simulink model "simulation_overall_1"  (R2024b)
settings: Solver=VariableStepAuto  StartTime=0.0  StopTime=10  MaxStep=1e-3  RelTol=1e-5
values from neighbouring files (symbols this model uses):
  dd_cable_len = diff(diff_cable_len)/dTheta    [sim_setup_1.m]
  del_theta = beam_defl    [sim_setup.m]    (also in sim_setup_1.m)
  del_theta0 = const.init_deflection    [sim_setup.m]    (also in sim_setup_1.m)
  diff_cable_len = diff(cable_len)/dTheta    [sim_setup_1.m]
  diff_del = diff(del_theta)/dTheta    [sim_setup.m]    (also in sim_setup_1.m)
  J = 0.0001    [sim_setup.m]    (also in sim_setup_1.m = 9.466956e-05)
  Jm = 32*1e-7    (= 3.2e-06)    [sim_setup_1.m]
  Jw = 12778*1e-9    (= 1.2778e-05)    [sim_setup_1.m]
  k = const.beam_stiffness    [sim_setup.m]    (also in sim_setup_1.m)
  Kt = 0.13    [sim_setup_1.m]
  N = 8    [sim_setup_1.m]
  R = 32e-3    (= 0.032)    [sim_setup_1.m]
  Sat_angle_max = ang(end)    [sim_setup_1.m]
  Sat_angle_min = ang(1)    [sim_setup_1.m]
  Sat_force_max = force(end)    [sim_setup_1.m]
  Sat_force_min = force(1)    [sim_setup_1.m]
  T_ang = ang(1:length(ang)-1)    [sim_setup.m]    (also in sim_setup_1.m)
undefined symbols (not defined in the file or in its folder): ang, cable_len
libraries: slpidlib x2, simulink_extras x1, simulink x1
settings Model: Creator=HNGG  LastModifiedBy=divg2
settings OptimizationCC: ReuseModelBlockBuffer=off
settings RTWCC: GPUComputeCapability=3.5

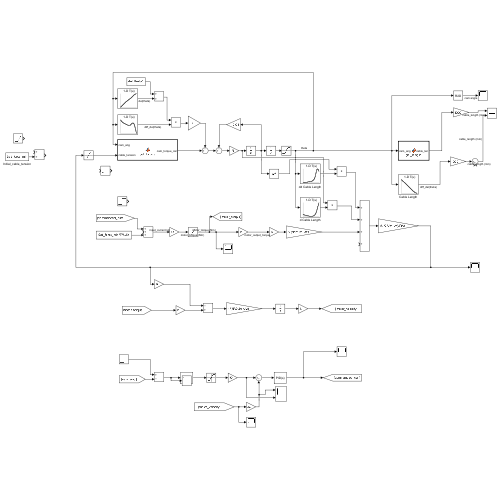
[thumbnail: Simulink's stored preview of the top-level diagram]
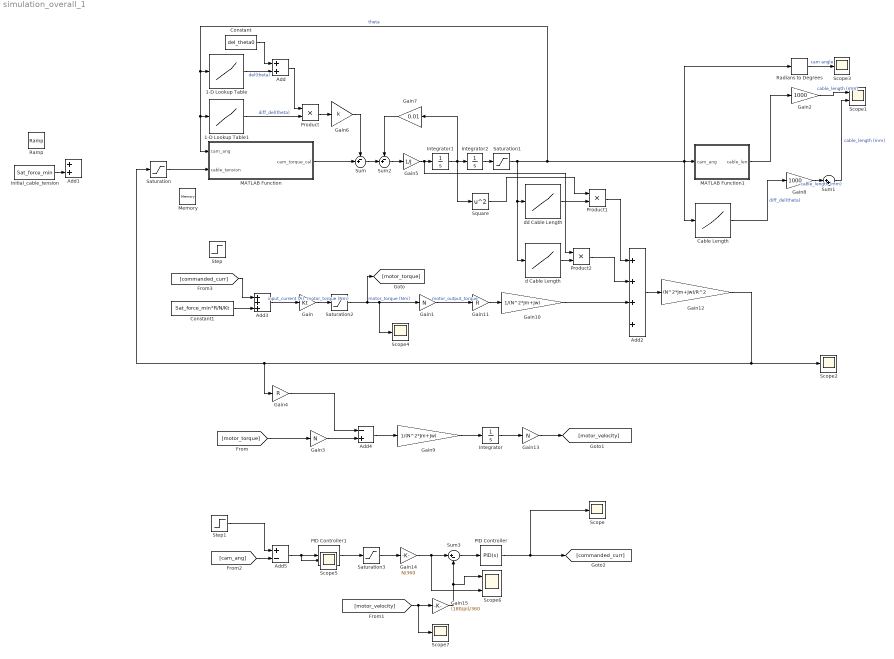
== system simulation_overall_1 ==
  1-D Lookup Table : Lookup_n-D  NumberOfTableDimensions=1  BreakpointsForDimension1=ang  Table=del_theta  InternalRulePriority=Speed  RndMeth=Simplest
  1-D Lookup Table1 : Lookup_n-D  NumberOfTableDimensions=1  BreakpointsForDimension1=T_ang  Table=diff_del  InternalRulePriority=Speed  RndMeth=Simplest
  Add : Sum
  Add1 : Sum
  Add2 : Sum  Inputs=++++
  Add3 : Sum  Inputs=+++
  Add4 : Sum  Inputs=-+
  Add5 : Sum  Inputs=+-
  Cable Length : Lookup_n-D  NumberOfTableDimensions=1  BreakpointsForDimension1=ang  Table=cable_len  InternalRulePriority=Speed  RndMeth=Simplest
  Constant : Constant  Value=del_theta0
  Constant1 : Constant  Value=Sat_force_min*R/N/Kt
  Gain : Gain  Gain=Kt
  Gain1 : Gain  Gain=N
  Gain10 : Gain  Gain=1/(N^2*Jm+Jw)
  Gain11 : Gain  Gain=R
  Gain12 : Gain  Gain=(N^2*Jm+Jw)/R^2
  Gain13 : Gain  Gain=N
  Gain14 : Gain  Gain=N/360
  Gain15 : Gain  Gain=(180/pi)/360
  Gain2 : Gain  Gain=1000
  Gain3 : Gain  Gain=N
  Gain4 : Gain  Gain=R
  Gain5 : Gain  Gain=1/J
  Gain6 : Gain  Gain=k
  Gain7 : Gain  Gain=0.01
  Gain8 : Gain  Gain=1000
  Gain9 : Gain  Gain=1/(N^2*Jm+Jw)
  Initial_cable_tension : Constant  Value=Sat_force_min
  Integrator : Integrator
  Integrator1 : Integrator
  Integrator2 : Integrator
  MATLAB Function : MATLAB Function  TreatAsAtomicUnit=on
  MATLAB Function1 : MATLAB Function  TreatAsAtomicUnit=on
  Memory : Memory  InitialCondition=Sat_force_min
  PID Controller : slpidlib/PID Controller  Controller=PID  Form=Parallel  TimeDomain=Continuous-time  UseExternalTs=off  SampleTime=-1  IntegratorMethod=Forward Euler  FilterMethod=Forward Euler  ControllerParametersSource=internal  P=4  I=1  UseKiTs=off  D=0.05  UseExternalDerivativeSource=off  N=100  UseFilter=on  TunerSelectOption=Transfer Function Based (PID Tuner App)  InitialConditionSource=internal  InitialConditionForIntegrator=0  InitialConditionForFilter=0  DifferentiatorICPrevScaledInput=0  ExternalReset=none  TrackingMode=off  Kt=1  LimitOutput=off  SatLimitsSource=internal  UpperSaturationLimit=inf  LowerSaturationLimit=-inf  LinearizeAsGain=on  AntiWindupMode=none  Kb=1  LimitIntegrator=off  UpperIntegratorSaturationLimit=inf  LowerIntegratorSaturationLimit=-inf  POutMin=[]  POutMax=[]  IOutMin=[]  IOutMax=[]  DOutMin=[]  DOutMax=[]  NOutMin=[]  NOutMax=[]  SumOutMin=[]  SumOutMax=[]  SaturationOutMin=[]  SaturationOutMax=[]  PParamMin=[]  PParamMax=[]  IParamMin=[]  IParamMax=[]  DParamMin=[]  DParamMax=[]  NParamMin=[]  NParamMax=[]  KbParamMin=[]  KbParamMax=[]  KtParamMin=[]  KtParamMax=[]  KbOutMin=[]  KbOutMax=[]  KtOutMin=[]  KtOutMax=[]  IntegratorOutMin=[]  IntegratorOutMax=[]  FilterOutMin=[]  FilterOutMax=[]  SumI1OutMin=[]  SumI1OutMax=[]  SumI2OutMin=[]  SumI2OutMax=[]  SumI3OutMin=[]  SumI3OutMax=[]  SumI4OutMin=[]  SumI4OutMax=[]  SumDOutMin=[]  SumDOutMax=[]  DifferentiatorOutMin=[]  DifferentiatorOutMax=[]  FilterDiffOutCoefMin=[]  FilterDiffOutCoefMax=[]  ReciprocalOutMin=[]  ReciprocalOutMax=[]  SumDenOutMin=[]  SumDenOutMax=[]  SumNumOutMin=[]  SumNumOutMax=[]  DivideOutMin=[]  DivideOutMax=[]  UdiffTsProdOutMin=[]  UdiffTsProdOutMax=[]  NTsProdOutMin=[]  NTsProdOutMax=[]  UintegralTsProdOutMin=[]  UintegralTsProdOutMax=[]  UngainTsProdOutMin=[]  UngainTsProdOutMax=[]  ClampingZeroOutDataTypeStr=Inherit: Inherit via back propagation  ClampingZeroOutMin=[]  ClampingZeroOutMax=[]  FilterDenConstantOutDataTypeStr=Inherit: Inherit via back propagation  FilterDenConstantOutMin=[]  FilterDenConstantOutMax=[]  PCopyOutDataTypeStr=Inherit: Inherit via back propagation  PCopyOutMin=[]  PCopyOutMax=[]  NCopyOutDataTypeStr=Inherit: Inherit via back propagation  NCopyOutMin=[]  NCopyOutMax=[]  IntegratorContinuousStateAttributes=''  IntegratorStateMustResolveToSignalObject=off  IntegratorRTWStateStorageClass=Auto  FilterContinuousStateAttributes=''  FilterStateMustResolveToSignalObject=off  FilterRTWStateStorageClass=Auto  ParallelPVariant=InternalParameters  IdealPVariant=Disabled  IVariant=InternalParameters  DVariant=InternalParameters  IntegratorVariant=Continuous  SatVariant=Disabled  AWVariant=Passthrough  PCopyVariant=Disabled  TRVariant=Disabled  FdbkBlocksVariant=Forward  IdealPFdbkVariant=Disabled  SatFdbkVariant=Disabled  DerivativeFilterVariant=ContFilter  NVariant=InternalParameters  NCopyVariant=Disabled  FilterICVariant=InternalICsFilter  IntegratorICVariant=InternalICs  ExternalResetVariant=Disabled  TRSumVariant=Passthrough  SumFdbkVariant=Disabled  SumVariant=Sum_PID  TsampFilterVariant=InternalTs  TsampNgainVariant=Passthrough  TsampIntegralVariant=Disabled_SignalSpec  ExternalSaturationOutDataTypeStr=Inherit: Same as second input  DerivativeSourceVariant=ErrorSignal  PreIntVariant=InternalPreInt
  PID Controller1 : slpidlib/PID Controller  Controller=PD  Form=Parallel  TimeDomain=Continuous-time  UseExternalTs=off  SampleTime=-1  IntegratorMethod=Forward Euler  FilterMethod=Forward Euler  ControllerParametersSource=internal  P=4  I=1  UseKiTs=off  D=0.01  UseExternalDerivativeSource=off  N=100  UseFilter=on  TunerSelectOption=Transfer Function Based (PID Tuner App)  InitialConditionSource=internal  InitialConditionForIntegrator=0  InitialConditionForFilter=0  DifferentiatorICPrevScaledInput=0  ExternalReset=none  TrackingMode=off  Kt=1  LimitOutput=off  SatLimitsSource=internal  UpperSaturationLimit=inf  LowerSaturationLimit=-inf  LinearizeAsGain=on  AntiWindupMode=none  Kb=1  LimitIntegrator=off  UpperIntegratorSaturationLimit=inf  LowerIntegratorSaturationLimit=-inf  POutMin=[]  POutMax=[]  IOutMin=[]  IOutMax=[]  DOutMin=[]  DOutMax=[]  NOutMin=[]  NOutMax=[]  SumOutMin=[]  SumOutMax=[]  SaturationOutMin=[]  SaturationOutMax=[]  PParamMin=[]  PParamMax=[]  IParamMin=[]  IParamMax=[]  DParamMin=[]  DParamMax=[]  NParamMin=[]  NParamMax=[]  KbParamMin=[]  KbParamMax=[]  KtParamMin=[]  KtParamMax=[]  KbOutMin=[]  KbOutMax=[]  KtOutMin=[]  KtOutMax=[]  IntegratorOutMin=[]  IntegratorOutMax=[]  FilterOutMin=[]  FilterOutMax=[]  SumI1OutMin=[]  SumI1OutMax=[]  SumI2OutMin=[]  SumI2OutMax=[]  SumI3OutMin=[]  SumI3OutMax=[]  SumI4OutMin=[]  SumI4OutMax=[]  SumDOutMin=[]  SumDOutMax=[]  DifferentiatorOutMin=[]  DifferentiatorOutMax=[]  FilterDiffOutCoefMin=[]  FilterDiffOutCoefMax=[]  ReciprocalOutMin=[]  ReciprocalOutMax=[]  SumDenOutMin=[]  SumDenOutMax=[]  SumNumOutMin=[]  SumNumOutMax=[]  DivideOutMin=[]  DivideOutMax=[]  UdiffTsProdOutMin=[]  UdiffTsProdOutMax=[]  NTsProdOutMin=[]  NTsProdOutMax=[]  UintegralTsProdOutMin=[]  UintegralTsProdOutMax=[]  UngainTsProdOutMin=[]  UngainTsProdOutMax=[]  ClampingZeroOutDataTypeStr=Inherit: Inherit via back propagation  ClampingZeroOutMin=[]  ClampingZeroOutMax=[]  FilterDenConstantOutDataTypeStr=Inherit: Inherit via back propagation  FilterDenConstantOutMin=[]  FilterDenConstantOutMax=[]  PCopyOutDataTypeStr=Inherit: Inherit via back propagation  PCopyOutMin=[]  PCopyOutMax=[]  NCopyOutDataTypeStr=Inherit: Inherit via back propagation  NCopyOutMin=[]  NCopyOutMax=[]  IntegratorContinuousStateAttributes=''  IntegratorStateMustResolveToSignalObject=off  IntegratorRTWStateStorageClass=Auto  FilterContinuousStateAttributes=''  FilterStateMustResolveToSignalObject=off  FilterRTWStateStorageClass=Auto  ParallelPVariant=InternalParameters  IdealPVariant=Disabled  IVariant=Disabled  DVariant=InternalParameters  IntegratorVariant=Disabled  SatVariant=Disabled  AWVariant=Disabled  PCopyVariant=Disabled  TRVariant=Disabled  FdbkBlocksVariant=Forward  IdealPFdbkVariant=Disabled  SatFdbkVariant=Disabled  DerivativeFilterVariant=ContFilter  NVariant=InternalParameters  NCopyVariant=Disabled  FilterICVariant=InternalICsFilter  IntegratorICVariant=Disabled  ExternalResetVariant=Disabled  TRSumVariant=Passthrough  SumFdbkVariant=Disabled  SumVariant=Sum_PD  TsampFilterVariant=InternalTs  TsampNgainVariant=Passthrough  TsampIntegralVariant=Disabled_SignalSpec  ExternalSaturationOutDataTypeStr=Inherit: Same as second input  DerivativeSourceVariant=ErrorSignal  PreIntVariant=InternalPreInt
  Product : Product
  Product1 : Product
  Product2 : Product
  Radians to Degrees : simulink_extras/Transformations/Radians to Degrees
  Ramp : simulink/Sources/Ramp  slope=1  start=2  InitialOutput=0
  Saturation : Saturate  UpperLimit=Sat_force_max  LowerLimit=Sat_force_min  ZeroCross=off
  Saturation1 : Saturate  UpperLimit=Sat_angle_max  LowerLimit=Sat_angle_min
  Saturation2 : Saturate  UpperLimit=5  LowerLimit=-5
  Saturation3 : Saturate  UpperLimit=4*360  LowerLimit=-4*360
  Scope{,2..5,7} (6 alike) : Scope
  Scope1 : Scope  NumInputPorts=2
  Scope6 : Scope  NumInputPorts=2
  Square : Math  Operator=square
  Step : Step  After=Sat_force_min*R/N/Kt*0.1  SampleTime=0
  Step1 : Step  Time=2  After=30  SampleTime=0
  Sum : Sum  Inputs=-+|
  Sum1 : Sum  Inputs=|++
  Sum2 : Sum  Inputs=-+|
  Sum3 : Sum  Inputs=|+-
  d Cable Length : Lookup_n-D  NumberOfTableDimensions=1  BreakpointsForDimension1=ang(1:end-1)  Table=diff_cable_len  InternalRulePriority=Speed  RndMeth=Simplest
  dd Cable Length : Lookup_n-D  NumberOfTableDimensions=1  BreakpointsForDimension1=ang(1:end-2)  Table=dd_cable_len  InternalRulePriority=Speed  RndMeth=Simplest
  wires:
  Gain12/1 -> Scope2/1, Gain4/1, Saturation/1
  Initial_cable_tension/1 -> Add1/2
  Add3/1 -> Gain/1  "input_current (A)"
  Saturation2/1 -> [motor_torque], Scope4/1, Gain1/1  "motor_torque (Nm)"
  Gain1/1 -> Gain11/1  "motor_output_torque"
  Radians to Degrees/1 -> Scope3/1  "cam angle"
  MATLAB Function1/1(cable_len) -> Gain2/1
  Gain2/1 -> Scope1/1  "cable_length (mm)"
  Constant/1 -> Add/1
  Product/1 -> Gain6/1
  Saturation1/1 -> d Cable Length/1, dd Cable Length/1, Radians to Degrees/1, Cable Length/1, MATLAB Function1/1(cam_ang), MATLAB Function/1(cam_ang), 1-D Lookup Table1/1, 1-D Lookup Table/1  "theta"
  Gain7/1 -> Sum2/1
  Add/1 -> Product/1
  Gain6/1 -> Sum/1
  Integrator2/1 -> Saturation1/1
  1-D Lookup Table/1 -> Add/2  "del(theta)"
  Gain5/1 -> Product2/1, Integrator1/1
  Sum/1 -> Sum2/2
  Sum2/1 -> Gain5/1
  MATLAB Function/1(cam_torque_cal) -> Sum/2
  1-D Lookup Table1/1 -> Product/2  "diff_del(theta)"
  Integrator1/1 -> Square/1, Gain7/1, Integrator2/1
  Cable Length/1 -> Gain8/1  "diff_del(theta)"
  Sum1/1 -> Scope1/2  "cable_length (mm)"
  Gain8/1 -> Sum1/1  "cable_length (mm)"
  Square/1 -> Product1/1
  Gain11/1 -> Gain10/1
  dd Cable Length/1 -> Product1/2
  d Cable Length/1 -> Product2/2
  Gain10/1 -> Add2/3
  Add2/1 -> Gain12/1
  Constant1/1 -> Add3/3
  Product2/1 -> Add2/2
  Product1/1 -> Add2/1
  Saturation/1 -> MATLAB Function/2(cable_tension)
  [motor_torque] -> Gain3/1
  Gain3/1 -> Add4/2
  Gain4/1 -> Add4/1
  Add4/1 -> Gain9/1
  Gain9/1 -> Integrator/1
  Integrator/1 -> Gain13/1
  Gain13/1 -> [motor_velocity]
  Add5/1 -> Scope5/1, PID Controller1/1
  Step1/1 -> Add5/1
  [cam_ang] -> Add5/2
  Sum3/1 -> PID Controller/1
  Saturation3/1 -> Gain14/1
  PID Controller1/1 -> Saturation3/1
  [motor_velocity] -> Scope7/1, Gain15/1
  Gain15/1 -> Sum3/2, Scope6/1
  PID Controller/1 -> Scope/1, [commanded_curr]
  Gain14/1 -> Scope6/2, Sum3/1
  [commanded_curr] -> Add3/1
  Gain/1 -> Saturation2/1  "motor_torque (Nm)"

== matlab function simulation_overall_1/MATLAB Function1 ==
  data: cam_ang input; cable_len output
function cable_len  = get_length(cam_ang)
lambda1 = pi/3;
lambda2 = pi/2;
r = 5/1000;
l_p3 = 55/1000;
P1 = [-23.61/1000; 18/1000; 0];
P2 = [-36.04/1000; 61.25/1000; 0];
theta = deg2rad(59)+cam_ang;
P3 = [l_p3*cos(theta); l_p3*sin(theta); 0];

d_13 = P1-P3;
d_23 = P2-P3;

beta1 = asin(2*r/norm(d_13));
beta2 = asin(2*r/norm(d_23));


% for P1
a1 = [0;-1;0]; b1 = -d_13;
psi1 = acos(dot(a1,b1)/norm(a1)/norm(b1));
cross1 = cross(a1,b1);
if cross1(3)<0
    psi1 = 2*pi - psi1;
end
wrapping_angle_p1 = 2*pi - lambda1 - (pi/2 - beta1) - psi1;
phi1 = -beta1+psi1;
r1 = r*[cos(phi1);sin(phi1);0];

% for P2
a2 = -d_23; b2 = [0;1;0];
psi2 = acos(dot(a2,b2)/norm(a2)/norm(b2));
cross2 = cross(a2,b2);
if cross2(3)<0
    psi2 = 2*pi - psi2;
end
wrapping_angle_p2 = 2*pi - lambda2 - (pi/2 - beta2) - psi2;
phi2 = beta2-psi2;
r2 = r*[cos(phi2);sin(phi2);0];

% for P3
% wrapping_angle_p3 = angle_between_two_vec(-r1,-r2);
a3 = -r1; b3 = -r2;
wrapping_angle_p3 = acos(dot(a3,b3)/norm(a3)/norm(b3));
cross3 = cross(a3,b3);
if cross3(3)<0
    wrapping_angle_p3 = 2*pi - wrapping_angle_p3;
end


% y1 = d_13 + 2*r1;
% tau1 = cable_tension*cross(P3-r1,y1/norm(y1));
% y2 = d_23 + 2*r2;
% tau2 = cable_tension*cross(P3-r2,y2/norm(y2));

% tau = tau1+tau2;
% cam_torque_cal = tau(3);

% cable lengths taut between pulleys
c1 = sqrt(norm(d_13)^2 - 4*r^2);
c2 = sqrt(norm(d_23)^2 - 4*r^2);
cable_len = c1 + c2 + (wrapping_angle_p1 + wrapping_angle_p2 + wrapping_angle_p3)*r;

end

== matlab function simulation_overall_1/MATLAB Function ==
  data: cam_ang input; cam_torque_cal output; cable_tension input
function cam_torque_cal  = get_torque(cam_ang,cable_tension)
% lambda1 = pi/3;
% lambda2 = pi/2;
r = 5/1000;
l_p3 = 55/1000;
P1 = [-23.61/1000; 18/1000; 0];
P2 = [-36.04/1000; 61.25/1000; 0];
theta = deg2rad(59)+cam_ang;
P3 = [l_p3*cos(theta); l_p3*sin(theta); 0];

d_13 = P1-P3;
d_23 = P2-P3;

beta1 = asin(2*r/norm(d_13));
beta2 = asin(2*r/norm(d_23));


% for P1
a1 = [0;-1;0]; b1 = -d_13;
psi1 = acos(dot(a1,b1)/norm(a1)/norm(b1));
cross1 = cross(a1,b1);
if cross1(3)<0
    psi1 = 2*pi - psi1;
end
% wrapping_angle_p1 = 2*pi - lambda1 - (pi/2 - beta1) - psi1;
phi1 = -beta1+psi1;
r1 = r*[cos(phi1);sin(phi1);0];

% for P2
a2 = -d_23; b2 = [0;1;0];
psi2 = acos(dot(a2,b2)/norm(a2)/norm(b2));
cross2 = cross(a2,b2);
if cross2(3)<0
    psi2 = 2*pi - psi2;
end
% wrapping_angle_p2 = 2*pi - lambda2 - (pi/2 - beta2) - psi2;
phi2 = beta2-psi2;
r2 = r*[cos(phi2);sin(phi2);0];

% for P3
% wrapping_angle_p3 = angle_between_two_vec(-r1,-r2);
% a3 = -r1; b3 = -r2;
% wrapping_angle_p3 = acos(dot(a3,b3)/norm(a3)/norm(b3));
% cross3 = cross(a3,b3);
% if cross3(3)<0
%     wrapping_angle_p3 = 2*pi - wrapping_angle_p3;
% end


y1 = d_13 + 2*r1;
tau1 = cable_tension*cross(P3-r1,y1/norm(y1));
y2 = d_23 + 2*r2;
tau2 = cable_tension*cross(P3-r2,y2/norm(y2));

tau = tau1+tau2;
cam_torque_cal = tau(3);

% cable lengths taut between pulleys
% c1 = sqrt(norm(d_13)^2 - 4*r^2);
% c2 = sqrt(norm(d_23)^2 - 4*r^2);
% cable_len = c1 + c2 + (wrapping_angle_p1 + wrapping_angle_p2 + wrapping_angle_p3)*r;

end
